simulink model "building_EXAMPLE_v1"  (R2016b)
settings: Solver=ode23tb  StartTime=-building.preruntime+8760*3600  StopTime=building.runtime+8760*3600  MaxStep=600  EnableMultiTasking=on
StartFcn:
  | tic
StopFcn:
  | toc
values from neighbouring files (symbols this model uses):
  building = create_building_automatic(building, modify, import_mode, name_XML, name_EXCEL, name_PHPP, NUMBEROFZONES)    [work_EXAMPLE_v1.m]
undefined symbols (not defined in the file or in its folder): A, B, C, cp, Dd, Dreifach, FluidMix, get_building, ID, MassFlow, p, Pressure, Qdot_C, Qdot_C_energy, Qdot_H, Qdot_H_energy, Qdot_I_electricity, Qdot_I_electricity_energy, Qdot_I_light, Qdot_I_light_energy, Qdot_I_person, Qdot_I_person_energy, Qdot_S, Qdot_S_energy, Qdot_T_ground, Qdot_T_ground_energy, Qdot_T_neighbour, Qdot_T_neighbour_energy, Qdot_T_opaque, Qdot_T_opaque_energy, Qdot_T_window, Qdot_T_window_energy, Qdot_V_infiltration, Qdot_V_infiltration_energy, Qdot_V_mech, Qdot_V_mech_energy, Qdot_V_window, Qdot_V_window_energy, rho, Tc, Temperature, Tr, Ts, Wärmeschutzglas, x_CO2, x_H2O, x_VOC
libraries: carnotUIBK x1931, carnot x83, simulink_extras x22, simulink x12
(part 13 of 35)

== system building_EXAMPLE_v1/HVAC pipes/ventilation_zone-to-zone 2-3 ==
  "[AIB]_in" : Inport
  "[AIB]_out" : Inport  Port=2
  Vdot : Inport  Port=3
  Bus Selector1 : BusSelector  OutputSignals=Tc,x_H2O,x_CO2,rho
  Bus Selector2 : BusSelector  OutputSignals=Tc,x_H2O,x_CO2,rho
  Demux5 : Demux  Outputs=2
  Fcn{1..4} (4 alike) : Fcn  Expr=u / (1+u)
  Gain : Gain  Gain=perc_Vdot_tot
  Gain{1,4..5,7} (4 alike) : Gain  Gain=-1
  Gain2 : Gain  Gain=0
  Ground{1..6,12..13} (8 alike) : Ground
  Mux1 : Mux  Inputs=[1 2 1 1 1 5 1 7]
  Mux2 : Mux  Inputs=[1 2 1 1 1 5 1 7]
  Mux3 : Mux  Inputs=2
  Mux6 : Mux  Inputs=2
  Product5 : Product  SaturateOnIntegerOverflow=on  InputSameDT=on  OutDataTypeStr=Inherit: Same as first input
  Product6 : Product  SaturateOnIntegerOverflow=on  InputSameDT=on  OutDataTypeStr=Inherit: Same as first input
  Product7 : Product  Inputs=3  SaturateOnIntegerOverflow=on  InputSameDT=on  OutDataTypeStr=Inherit: Same as first input
  Sum1 : Sum  Inputs=-+  SaturateOnIntegerOverflow=on  InputSameDT=on  OutDataTypeStr=Inherit: Same as first input
  Switch : Switch  Criteria=u2 > Threshold
  Switch1 : Switch  Criteria=u2 > Threshold
  cp : Constant  Value=1006.8
  h/s : Gain  Gain=1/3600
  "[S]_in" : Outport
  "[S]_out" : Outport  Port=2
  wires:
  Mux3/1 -> Switch1/1
  Mux6/1 -> Switch1/3
  Bus Selector1/3 -> Fcn3/1  "<x_CO2>"
  Bus Selector1/2 -> Fcn4/1  "<x_H2O>"
  Fcn3/1 -> Mux3/2
  Fcn4/1 -> Mux3/1
  Bus Selector2/4 -> Switch/3  "<rho>"
  Bus Selector1/4 -> Switch/1  "<rho>"
  "[AIB]_in"/1 -> Bus Selector1/1
  cp/1 -> Product7/3
  Ground4/1 -> Mux1/7
  Ground1/1 -> Mux1/8
  "[AIB]_out"/1 -> Bus Selector2/1
  Bus Selector1/1 -> Sum1/1  "<Tc>"
  Fcn1/1 -> Mux6/2
  Fcn2/1 -> Mux6/1
  Ground12/1 -> Mux1/6
  Product5/1 -> Demux5/1
  Bus Selector2/3 -> Fcn1/1  "<x_CO2>"
  Mux2/1 -> "[S]_out"/1
  Switch/1 -> Product6/2  "rho"
  Product6/1 -> Gain1/1
  Gain/1 -> Switch/2, Switch1/2, h/s/1
  Mux1/1 -> "[S]_in"/1
  Product7/1 -> Gain2/1, Mux1/1  "Qdot_air"
  Ground13/1 -> Mux1/2
  Demux5/2 -> Mux1/5, Gain5/1  "mdot_CO2"
  Demux5/1 -> Mux1/4, Gain4/1  "mdot_H2O"
  Bus Selector2/1 -> Sum1/2  "<Tc>"
  Bus Selector2/2 -> Fcn2/1  "<x_H2O>"
  Switch1/1 -> Product5/2
  Sum1/1 -> Product7/1  "dT"
  Vdot/1 -> Gain/1
  h/s/1 -> Product6/1
  Gain1/1 -> Gain7/1, Product5/1, Product7/2, Mux1/3  "massflow"
  Ground3/1 -> Mux2/7
  Gain4/1 -> Mux2/4
  Gain7/1 -> Mux2/3
  Ground2/1 -> Mux2/2
  Gain5/1 -> Mux2/5
  Ground5/1 -> Mux2/6
  Ground6/1 -> Mux2/8
  Gain2/1 -> Mux2/1

== system building_EXAMPLE_v1/HVAC pipes/ventilation_zone-to-zone 2-4 ==
  "[AIB]_in" : Inport
  "[AIB]_out" : Inport  Port=2
  Vdot : Inport  Port=3
  Bus Selector1 : BusSelector  OutputSignals=Tc,x_H2O,x_CO2,rho
  Bus Selector2 : BusSelector  OutputSignals=Tc,x_H2O,x_CO2,rho
  Demux5 : Demux  Outputs=2
  Fcn{1..4} (4 alike) : Fcn  Expr=u / (1+u)
  Gain : Gain  Gain=perc_Vdot_tot
  Gain{1,4..5,7} (4 alike) : Gain  Gain=-1
  Gain2 : Gain  Gain=0
  Ground{1..6,12..13} (8 alike) : Ground
  Mux1 : Mux  Inputs=[1 2 1 1 1 5 1 7]
  Mux2 : Mux  Inputs=[1 2 1 1 1 5 1 7]
  Mux3 : Mux  Inputs=2
  Mux6 : Mux  Inputs=2
  Product5 : Product  SaturateOnIntegerOverflow=on  InputSameDT=on  OutDataTypeStr=Inherit: Same as first input
  Product6 : Product  SaturateOnIntegerOverflow=on  InputSameDT=on  OutDataTypeStr=Inherit: Same as first input
  Product7 : Product  Inputs=3  SaturateOnIntegerOverflow=on  InputSameDT=on  OutDataTypeStr=Inherit: Same as first input
  Sum1 : Sum  Inputs=-+  SaturateOnIntegerOverflow=on  InputSameDT=on  OutDataTypeStr=Inherit: Same as first input
  Switch : Switch  Criteria=u2 > Threshold
  Switch1 : Switch  Criteria=u2 > Threshold
  cp : Constant  Value=1006.8
  h/s : Gain  Gain=1/3600
  "[S]_in" : Outport
  "[S]_out" : Outport  Port=2
  wires:
  Mux3/1 -> Switch1/1
  Mux6/1 -> Switch1/3
  Bus Selector1/3 -> Fcn3/1  "<x_CO2>"
  Bus Selector1/2 -> Fcn4/1  "<x_H2O>"
  Fcn3/1 -> Mux3/2
  Fcn4/1 -> Mux3/1
  Bus Selector2/4 -> Switch/3  "<rho>"
  Bus Selector1/4 -> Switch/1  "<rho>"
  "[AIB]_in"/1 -> Bus Selector1/1
  cp/1 -> Product7/3
  Ground4/1 -> Mux1/7
  Ground1/1 -> Mux1/8
  "[AIB]_out"/1 -> Bus Selector2/1
  Bus Selector1/1 -> Sum1/1  "<Tc>"
  Fcn1/1 -> Mux6/2
  Fcn2/1 -> Mux6/1
  Ground12/1 -> Mux1/6
  Product5/1 -> Demux5/1
  Bus Selector2/3 -> Fcn1/1  "<x_CO2>"
  Mux2/1 -> "[S]_out"/1
  Switch/1 -> Product6/2  "rho"
  Product6/1 -> Gain1/1
  Gain/1 -> Switch/2, Switch1/2, h/s/1
  Mux1/1 -> "[S]_in"/1
  Product7/1 -> Gain2/1, Mux1/1  "Qdot_air"
  Ground13/1 -> Mux1/2
  Demux5/2 -> Mux1/5, Gain5/1  "mdot_CO2"
  Demux5/1 -> Mux1/4, Gain4/1  "mdot_H2O"
  Bus Selector2/1 -> Sum1/2  "<Tc>"
  Bus Selector2/2 -> Fcn2/1  "<x_H2O>"
  Switch1/1 -> Product5/2
  Sum1/1 -> Product7/1  "dT"
  Vdot/1 -> Gain/1
  h/s/1 -> Product6/1
  Gain1/1 -> Gain7/1, Product5/1, Product7/2, Mux1/3  "massflow"
  Ground3/1 -> Mux2/7
  Gain4/1 -> Mux2/4
  Gain7/1 -> Mux2/3
  Ground2/1 -> Mux2/2
  Gain5/1 -> Mux2/5
  Ground5/1 -> Mux2/6
  Ground6/1 -> Mux2/8
  Gain2/1 -> Mux2/1

== system building_EXAMPLE_v1/HVAC pipes/ventilation_zone-to-zone 2-5 ==
  "[AIB]_in" : Inport
  "[AIB]_out" : Inport  Port=2
  Vdot : Inport  Port=3
  Bus Selector1 : BusSelector  OutputSignals=Tc,x_H2O,x_CO2,rho
  Bus Selector2 : BusSelector  OutputSignals=Tc,x_H2O,x_CO2,rho
  Demux5 : Demux  Outputs=2
  Fcn{1..4} (4 alike) : Fcn  Expr=u / (1+u)
  Gain : Gain  Gain=perc_Vdot_tot
  Gain{1,4..5,7} (4 alike) : Gain  Gain=-1
  Gain2 : Gain  Gain=0
  Ground{1..6,12..13} (8 alike) : Ground
  Mux1 : Mux  Inputs=[1 2 1 1 1 5 1 7]
  Mux2 : Mux  Inputs=[1 2 1 1 1 5 1 7]
  Mux3 : Mux  Inputs=2
  Mux6 : Mux  Inputs=2
  Product5 : Product  SaturateOnIntegerOverflow=on  InputSameDT=on  OutDataTypeStr=Inherit: Same as first input
  Product6 : Product  SaturateOnIntegerOverflow=on  InputSameDT=on  OutDataTypeStr=Inherit: Same as first input
  Product7 : Product  Inputs=3  SaturateOnIntegerOverflow=on  InputSameDT=on  OutDataTypeStr=Inherit: Same as first input
  Sum1 : Sum  Inputs=-+  SaturateOnIntegerOverflow=on  InputSameDT=on  OutDataTypeStr=Inherit: Same as first input
  Switch : Switch  Criteria=u2 > Threshold
  Switch1 : Switch  Criteria=u2 > Threshold
  cp : Constant  Value=1006.8
  h/s : Gain  Gain=1/3600
  "[S]_in" : Outport
  "[S]_out" : Outport  Port=2
  wires:
  Mux3/1 -> Switch1/1
  Mux6/1 -> Switch1/3
  Bus Selector1/3 -> Fcn3/1  "<x_CO2>"
  Bus Selector1/2 -> Fcn4/1  "<x_H2O>"
  Fcn3/1 -> Mux3/2
  Fcn4/1 -> Mux3/1
  Bus Selector2/4 -> Switch/3  "<rho>"
  Bus Selector1/4 -> Switch/1  "<rho>"
  "[AIB]_in"/1 -> Bus Selector1/1
  cp/1 -> Product7/3
  Ground4/1 -> Mux1/7
  Ground1/1 -> Mux1/8
  "[AIB]_out"/1 -> Bus Selector2/1
  Bus Selector1/1 -> Sum1/1  "<Tc>"
  Fcn1/1 -> Mux6/2
  Fcn2/1 -> Mux6/1
  Ground12/1 -> Mux1/6
  Product5/1 -> Demux5/1
  Bus Selector2/3 -> Fcn1/1  "<x_CO2>"
  Mux2/1 -> "[S]_out"/1
  Switch/1 -> Product6/2  "rho"
  Product6/1 -> Gain1/1
  Gain/1 -> Switch/2, Switch1/2, h/s/1
  Mux1/1 -> "[S]_in"/1
  Product7/1 -> Gain2/1, Mux1/1  "Qdot_air"
  Ground13/1 -> Mux1/2
  Demux5/2 -> Mux1/5, Gain5/1  "mdot_CO2"
  Demux5/1 -> Mux1/4, Gain4/1  "mdot_H2O"
  Bus Selector2/1 -> Sum1/2  "<Tc>"
  Bus Selector2/2 -> Fcn2/1  "<x_H2O>"
  Switch1/1 -> Product5/2
  Sum1/1 -> Product7/1  "dT"
  Vdot/1 -> Gain/1
  h/s/1 -> Product6/1
  Gain1/1 -> Gain7/1, Product5/1, Product7/2, Mux1/3  "massflow"
  Ground3/1 -> Mux2/7
  Gain4/1 -> Mux2/4
  Gain7/1 -> Mux2/3
  Ground2/1 -> Mux2/2
  Gain5/1 -> Mux2/5
  Ground5/1 -> Mux2/6
  Ground6/1 -> Mux2/8
  Gain2/1 -> Mux2/1

== system building_EXAMPLE_v1/HVAC pipes/ventilation_zone-to-zone 2-6 ==
  "[AIB]_in" : Inport
  "[AIB]_out" : Inport  Port=2
  Vdot : Inport  Port=3
  Bus Selector1 : BusSelector  OutputSignals=Tc,x_H2O,x_CO2,rho
  Bus Selector2 : BusSelector  OutputSignals=Tc,x_H2O,x_CO2,rho
  Demux5 : Demux  Outputs=2
  Fcn{1..4} (4 alike) : Fcn  Expr=u / (1+u)
  Gain : Gain  Gain=perc_Vdot_tot
  Gain{1,4..5,7} (4 alike) : Gain  Gain=-1
  Gain2 : Gain  Gain=0
  Ground{1..6,12..13} (8 alike) : Ground
  Mux1 : Mux  Inputs=[1 2 1 1 1 5 1 7]
  Mux2 : Mux  Inputs=[1 2 1 1 1 5 1 7]
  Mux3 : Mux  Inputs=2
  Mux6 : Mux  Inputs=2
  Product5 : Product  SaturateOnIntegerOverflow=on  InputSameDT=on  OutDataTypeStr=Inherit: Same as first input
  Product6 : Product  SaturateOnIntegerOverflow=on  InputSameDT=on  OutDataTypeStr=Inherit: Same as first input
  Product7 : Product  Inputs=3  SaturateOnIntegerOverflow=on  InputSameDT=on  OutDataTypeStr=Inherit: Same as first input
  Sum1 : Sum  Inputs=-+  SaturateOnIntegerOverflow=on  InputSameDT=on  OutDataTypeStr=Inherit: Same as first input
  Switch : Switch  Criteria=u2 > Threshold
  Switch1 : Switch  Criteria=u2 > Threshold
  cp : Constant  Value=1006.8
  h/s : Gain  Gain=1/3600
  "[S]_in" : Outport
  "[S]_out" : Outport  Port=2
  wires:
  Mux3/1 -> Switch1/1
  Mux6/1 -> Switch1/3
  Bus Selector1/3 -> Fcn3/1  "<x_CO2>"
  Bus Selector1/2 -> Fcn4/1  "<x_H2O>"
  Fcn3/1 -> Mux3/2
  Fcn4/1 -> Mux3/1
  Bus Selector2/4 -> Switch/3  "<rho>"
  Bus Selector1/4 -> Switch/1  "<rho>"
  "[AIB]_in"/1 -> Bus Selector1/1
  cp/1 -> Product7/3
  Ground4/1 -> Mux1/7
  Ground1/1 -> Mux1/8
  "[AIB]_out"/1 -> Bus Selector2/1
  Bus Selector1/1 -> Sum1/1  "<Tc>"
  Fcn1/1 -> Mux6/2
  Fcn2/1 -> Mux6/1
  Ground12/1 -> Mux1/6
  Product5/1 -> Demux5/1
  Bus Selector2/3 -> Fcn1/1  "<x_CO2>"
  Mux2/1 -> "[S]_out"/1
  Switch/1 -> Product6/2  "rho"
  Product6/1 -> Gain1/1
  Gain/1 -> Switch/2, Switch1/2, h/s/1
  Mux1/1 -> "[S]_in"/1
  Product7/1 -> Gain2/1, Mux1/1  "Qdot_air"
  Ground13/1 -> Mux1/2
  Demux5/2 -> Mux1/5, Gain5/1  "mdot_CO2"
  Demux5/1 -> Mux1/4, Gain4/1  "mdot_H2O"
  Bus Selector2/1 -> Sum1/2  "<Tc>"
  Bus Selector2/2 -> Fcn2/1  "<x_H2O>"
  Switch1/1 -> Product5/2
  Sum1/1 -> Product7/1  "dT"
  Vdot/1 -> Gain/1
  h/s/1 -> Product6/1
  Gain1/1 -> Gain7/1, Product5/1, Product7/2, Mux1/3  "massflow"
  Ground3/1 -> Mux2/7
  Gain4/1 -> Mux2/4
  Gain7/1 -> Mux2/3
  Ground2/1 -> Mux2/2
  Gain5/1 -> Mux2/5
  Ground5/1 -> Mux2/6
  Ground6/1 -> Mux2/8
  Gain2/1 -> Mux2/1

== system building_EXAMPLE_v1/HVAC pipes/ventilation_zone-to-zone 2-7 ==
  "[AIB]_in" : Inport
  "[AIB]_out" : Inport  Port=2
  Vdot : Inport  Port=3
  Bus Selector1 : BusSelector  OutputSignals=Tc,x_H2O,x_CO2,rho
  Bus Selector2 : BusSelector  OutputSignals=Tc,x_H2O,x_CO2,rho
  Demux5 : Demux  Outputs=2
  Fcn{1..4} (4 alike) : Fcn  Expr=u / (1+u)
  Gain : Gain  Gain=perc_Vdot_tot
  Gain{1,4..5,7} (4 alike) : Gain  Gain=-1
  Gain2 : Gain  Gain=0
  Ground{1..6,12..13} (8 alike) : Ground
  Mux1 : Mux  Inputs=[1 2 1 1 1 5 1 7]
  Mux2 : Mux  Inputs=[1 2 1 1 1 5 1 7]
  Mux3 : Mux  Inputs=2
  Mux6 : Mux  Inputs=2
  Product5 : Product  SaturateOnIntegerOverflow=on  InputSameDT=on  OutDataTypeStr=Inherit: Same as first input
  Product6 : Product  SaturateOnIntegerOverflow=on  InputSameDT=on  OutDataTypeStr=Inherit: Same as first input
  Product7 : Product  Inputs=3  SaturateOnIntegerOverflow=on  InputSameDT=on  OutDataTypeStr=Inherit: Same as first input
  Sum1 : Sum  Inputs=-+  SaturateOnIntegerOverflow=on  InputSameDT=on  OutDataTypeStr=Inherit: Same as first input
  Switch : Switch  Criteria=u2 > Threshold
  Switch1 : Switch  Criteria=u2 > Threshold
  cp : Constant  Value=1006.8
  h/s : Gain  Gain=1/3600
  "[S]_in" : Outport
  "[S]_out" : Outport  Port=2
  wires:
  Mux3/1 -> Switch1/1
  Mux6/1 -> Switch1/3
  Bus Selector1/3 -> Fcn3/1  "<x_CO2>"
  Bus Selector1/2 -> Fcn4/1  "<x_H2O>"
  Fcn3/1 -> Mux3/2
  Fcn4/1 -> Mux3/1
  Bus Selector2/4 -> Switch/3  "<rho>"
  Bus Selector1/4 -> Switch/1  "<rho>"
  "[AIB]_in"/1 -> Bus Selector1/1
  cp/1 -> Product7/3
  Ground4/1 -> Mux1/7
  Ground1/1 -> Mux1/8
  "[AIB]_out"/1 -> Bus Selector2/1
  Bus Selector1/1 -> Sum1/1  "<Tc>"
  Fcn1/1 -> Mux6/2
  Fcn2/1 -> Mux6/1
  Ground12/1 -> Mux1/6
  Product5/1 -> Demux5/1
  Bus Selector2/3 -> Fcn1/1  "<x_CO2>"
  Mux2/1 -> "[S]_out"/1
  Switch/1 -> Product6/2  "rho"
  Product6/1 -> Gain1/1
  Gain/1 -> Switch/2, Switch1/2, h/s/1
  Mux1/1 -> "[S]_in"/1
  Product7/1 -> Gain2/1, Mux1/1  "Qdot_air"
  Ground13/1 -> Mux1/2
  Demux5/2 -> Mux1/5, Gain5/1  "mdot_CO2"
  Demux5/1 -> Mux1/4, Gain4/1  "mdot_H2O"
  Bus Selector2/1 -> Sum1/2  "<Tc>"
  Bus Selector2/2 -> Fcn2/1  "<x_H2O>"
  Switch1/1 -> Product5/2
  Sum1/1 -> Product7/1  "dT"
  Vdot/1 -> Gain/1
  h/s/1 -> Product6/1
  Gain1/1 -> Gain7/1, Product5/1, Product7/2, Mux1/3  "massflow"
  Ground3/1 -> Mux2/7
  Gain4/1 -> Mux2/4
  Gain7/1 -> Mux2/3
  Ground2/1 -> Mux2/2
  Gain5/1 -> Mux2/5
  Ground5/1 -> Mux2/6
  Ground6/1 -> Mux2/8
  Gain2/1 -> Mux2/1

== system building_EXAMPLE_v1/HVAC pipes/ventilation_zone-to-zone 2-8 ==
  "[AIB]_in" : Inport
  "[AIB]_out" : Inport  Port=2
  Vdot : Inport  Port=3
  Bus Selector1 : BusSelector  OutputSignals=Tc,x_H2O,x_CO2,rho
  Bus Selector2 : BusSelector  OutputSignals=Tc,x_H2O,x_CO2,rho
  Demux5 : Demux  Outputs=2
  Fcn{1..4} (4 alike) : Fcn  Expr=u / (1+u)
  Gain : Gain  Gain=perc_Vdot_tot
  Gain{1,4..5,7} (4 alike) : Gain  Gain=-1
  Gain2 : Gain  Gain=0
  Ground{1..6,12..13} (8 alike) : Ground
  Mux1 : Mux  Inputs=[1 2 1 1 1 5 1 7]
  Mux2 : Mux  Inputs=[1 2 1 1 1 5 1 7]
  Mux3 : Mux  Inputs=2
  Mux6 : Mux  Inputs=2
  Product5 : Product  SaturateOnIntegerOverflow=on  InputSameDT=on  OutDataTypeStr=Inherit: Same as first input
  Product6 : Product  SaturateOnIntegerOverflow=on  InputSameDT=on  OutDataTypeStr=Inherit: Same as first input
  Product7 : Product  Inputs=3  SaturateOnIntegerOverflow=on  InputSameDT=on  OutDataTypeStr=Inherit: Same as first input
  Sum1 : Sum  Inputs=-+  SaturateOnIntegerOverflow=on  InputSameDT=on  OutDataTypeStr=Inherit: Same as first input
  Switch : Switch  Criteria=u2 > Threshold
  Switch1 : Switch  Criteria=u2 > Threshold
  cp : Constant  Value=1006.8
  h/s : Gain  Gain=1/3600
  "[S]_in" : Outport
  "[S]_out" : Outport  Port=2
  wires:
  Mux3/1 -> Switch1/1
  Mux6/1 -> Switch1/3
  Bus Selector1/3 -> Fcn3/1  "<x_CO2>"
  Bus Selector1/2 -> Fcn4/1  "<x_H2O>"
  Fcn3/1 -> Mux3/2
  Fcn4/1 -> Mux3/1
  Bus Selector2/4 -> Switch/3  "<rho>"
  Bus Selector1/4 -> Switch/1  "<rho>"
  "[AIB]_in"/1 -> Bus Selector1/1
  cp/1 -> Product7/3
  Ground4/1 -> Mux1/7
  Ground1/1 -> Mux1/8
  "[AIB]_out"/1 -> Bus Selector2/1
  Bus Selector1/1 -> Sum1/1  "<Tc>"
  Fcn1/1 -> Mux6/2
  Fcn2/1 -> Mux6/1
  Ground12/1 -> Mux1/6
  Product5/1 -> Demux5/1
  Bus Selector2/3 -> Fcn1/1  "<x_CO2>"
  Mux2/1 -> "[S]_out"/1
  Switch/1 -> Product6/2  "rho"
  Product6/1 -> Gain1/1
  Gain/1 -> Switch/2, Switch1/2, h/s/1
  Mux1/1 -> "[S]_in"/1
  Product7/1 -> Gain2/1, Mux1/1  "Qdot_air"
  Ground13/1 -> Mux1/2
  Demux5/2 -> Mux1/5, Gain5/1  "mdot_CO2"
  Demux5/1 -> Mux1/4, Gain4/1  "mdot_H2O"
  Bus Selector2/1 -> Sum1/2  "<Tc>"
  Bus Selector2/2 -> Fcn2/1  "<x_H2O>"
  Switch1/1 -> Product5/2
  Sum1/1 -> Product7/1  "dT"
  Vdot/1 -> Gain/1
  h/s/1 -> Product6/1
  Gain1/1 -> Gain7/1, Product5/1, Product7/2, Mux1/3  "massflow"
  Ground3/1 -> Mux2/7
  Gain4/1 -> Mux2/4
  Gain7/1 -> Mux2/3
  Ground2/1 -> Mux2/2
  Gain5/1 -> Mux2/5
  Ground5/1 -> Mux2/6
  Ground6/1 -> Mux2/8
  Gain2/1 -> Mux2/1

== system building_EXAMPLE_v1/HVAC pipes/ventilation_zone-to-zone 2-9 ==
  "[AIB]_in" : Inport
  "[AIB]_out" : Inport  Port=2
  Vdot : Inport  Port=3
  Bus Selector1 : BusSelector  OutputSignals=Tc,x_H2O,x_CO2,rho
  Bus Selector2 : BusSelector  OutputSignals=Tc,x_H2O,x_CO2,rho
  Demux5 : Demux  Outputs=2
  Fcn{1..4} (4 alike) : Fcn  Expr=u / (1+u)
  Gain : Gain  Gain=perc_Vdot_tot
  Gain{1,4..5,7} (4 alike) : Gain  Gain=-1
  Gain2 : Gain  Gain=0
  Ground{1..6,12..13} (8 alike) : Ground
  Mux1 : Mux  Inputs=[1 2 1 1 1 5 1 7]
  Mux2 : Mux  Inputs=[1 2 1 1 1 5 1 7]
  Mux3 : Mux  Inputs=2
  Mux6 : Mux  Inputs=2
  Product5 : Product  SaturateOnIntegerOverflow=on  InputSameDT=on  OutDataTypeStr=Inherit: Same as first input
  Product6 : Product  SaturateOnIntegerOverflow=on  InputSameDT=on  OutDataTypeStr=Inherit: Same as first input
  Product7 : Product  Inputs=3  SaturateOnIntegerOverflow=on  InputSameDT=on  OutDataTypeStr=Inherit: Same as first input
  Sum1 : Sum  Inputs=-+  SaturateOnIntegerOverflow=on  InputSameDT=on  OutDataTypeStr=Inherit: Same as first input
  Switch : Switch  Criteria=u2 > Threshold
  Switch1 : Switch  Criteria=u2 > Threshold
  cp : Constant  Value=1006.8
  h/s : Gain  Gain=1/3600
  "[S]_in" : Outport
  "[S]_out" : Outport  Port=2
  wires:
  Mux3/1 -> Switch1/1
  Mux6/1 -> Switch1/3
  Bus Selector1/3 -> Fcn3/1  "<x_CO2>"
  Bus Selector1/2 -> Fcn4/1  "<x_H2O>"
  Fcn3/1 -> Mux3/2
  Fcn4/1 -> Mux3/1
  Bus Selector2/4 -> Switch/3  "<rho>"
  Bus Selector1/4 -> Switch/1  "<rho>"
  "[AIB]_in"/1 -> Bus Selector1/1
  cp/1 -> Product7/3
  Ground4/1 -> Mux1/7
  Ground1/1 -> Mux1/8
  "[AIB]_out"/1 -> Bus Selector2/1
  Bus Selector1/1 -> Sum1/1  "<Tc>"
  Fcn1/1 -> Mux6/2
  Fcn2/1 -> Mux6/1
  Ground12/1 -> Mux1/6
  Product5/1 -> Demux5/1
  Bus Selector2/3 -> Fcn1/1  "<x_CO2>"
  Mux2/1 -> "[S]_out"/1
  Switch/1 -> Product6/2  "rho"
  Product6/1 -> Gain1/1
  Gain/1 -> Switch/2, Switch1/2, h/s/1
  Mux1/1 -> "[S]_in"/1
  Product7/1 -> Gain2/1, Mux1/1  "Qdot_air"
  Ground13/1 -> Mux1/2
  Demux5/2 -> Mux1/5, Gain5/1  "mdot_CO2"
  Demux5/1 -> Mux1/4, Gain4/1  "mdot_H2O"
  Bus Selector2/1 -> Sum1/2  "<Tc>"
  Bus Selector2/2 -> Fcn2/1  "<x_H2O>"
  Switch1/1 -> Product5/2
  Sum1/1 -> Product7/1  "dT"
  Vdot/1 -> Gain/1
  h/s/1 -> Product6/1
  Gain1/1 -> Gain7/1, Product5/1, Product7/2, Mux1/3  "massflow"
  Ground3/1 -> Mux2/7
  Gain4/1 -> Mux2/4
  Gain7/1 -> Mux2/3
  Ground2/1 -> Mux2/2
  Gain5/1 -> Mux2/5
  Ground5/1 -> Mux2/6
  Ground6/1 -> Mux2/8
  Gain2/1 -> Mux2/1

== system building_EXAMPLE_v1/HVAC pipes/ventilation_zone-to-zone 3-10 ==
  "[AIB]_in" : Inport
  "[AIB]_out" : Inport  Port=2
  Vdot : Inport  Port=3
  Bus Selector1 : BusSelector  OutputSignals=Tc,x_H2O,x_CO2,rho
  Bus Selector2 : BusSelector  OutputSignals=Tc,x_H2O,x_CO2,rho
  Demux5 : Demux  Outputs=2
  Fcn{1..4} (4 alike) : Fcn  Expr=u / (1+u)
  Gain : Gain  Gain=perc_Vdot_tot
  Gain{1,4..5,7} (4 alike) : Gain  Gain=-1
  Gain2 : Gain  Gain=0
  Ground{1..6,12..13} (8 alike) : Ground
  Mux1 : Mux  Inputs=[1 2 1 1 1 5 1 7]
  Mux2 : Mux  Inputs=[1 2 1 1 1 5 1 7]
  Mux3 : Mux  Inputs=2
  Mux6 : Mux  Inputs=2
  Product5 : Product  SaturateOnIntegerOverflow=on  InputSameDT=on  OutDataTypeStr=Inherit: Same as first input
  Product6 : Product  SaturateOnIntegerOverflow=on  InputSameDT=on  OutDataTypeStr=Inherit: Same as first input
  Product7 : Product  Inputs=3  SaturateOnIntegerOverflow=on  InputSameDT=on  OutDataTypeStr=Inherit: Same as first input
  Sum1 : Sum  Inputs=-+  SaturateOnIntegerOverflow=on  InputSameDT=on  OutDataTypeStr=Inherit: Same as first input
  Switch : Switch  Criteria=u2 > Threshold
  Switch1 : Switch  Criteria=u2 > Threshold
  cp : Constant  Value=1006.8
  h/s : Gain  Gain=1/3600
  "[S]_in" : Outport
  "[S]_out" : Outport  Port=2
  wires:
  Gain2/1 -> Mux2/1
  Ground6/1 -> Mux2/8
  Ground5/1 -> Mux2/6
  Gain5/1 -> Mux2/5
  Ground2/1 -> Mux2/2
  Gain7/1 -> Mux2/3
  Gain4/1 -> Mux2/4
  Ground3/1 -> Mux2/7
  Gain1/1 -> Mux1/3, Product7/2, Product5/1, Gain7/1  "massflow"
  h/s/1 -> Product6/1
  Vdot/1 -> Gain/1
  Sum1/1 -> Product7/1  "dT"
  Switch1/1 -> Product5/2
  Bus Selector2/2 -> Fcn2/1  "<x_H2O>"
  Bus Selector2/1 -> Sum1/2  "<Tc>"
  Demux5/1 -> Gain4/1, Mux1/4  "mdot_H2O"
  Demux5/2 -> Gain5/1, Mux1/5  "mdot_CO2"
  Ground13/1 -> Mux1/2
  Product7/1 -> Mux1/1, Gain2/1  "Qdot_air"
  Mux1/1 -> "[S]_in"/1
  Gain/1 -> h/s/1, Switch1/2, Switch/2
  Product6/1 -> Gain1/1
  Switch/1 -> Product6/2  "rho"
  Mux2/1 -> "[S]_out"/1
  Bus Selector2/3 -> Fcn1/1  "<x_CO2>"
  Product5/1 -> Demux5/1
  Ground12/1 -> Mux1/6
  Fcn2/1 -> Mux6/1
  Fcn1/1 -> Mux6/2
  Bus Selector1/1 -> Sum1/1  "<Tc>"
  "[AIB]_out"/1 -> Bus Selector2/1
  Ground1/1 -> Mux1/8
  Ground4/1 -> Mux1/7
  cp/1 -> Product7/3
  "[AIB]_in"/1 -> Bus Selector1/1
  Bus Selector1/4 -> Switch/1  "<rho>"
  Bus Selector2/4 -> Switch/3  "<rho>"
  Fcn4/1 -> Mux3/1
  Fcn3/1 -> Mux3/2
  Bus Selector1/2 -> Fcn4/1  "<x_H2O>"
  Bus Selector1/3 -> Fcn3/1  "<x_CO2>"
  Mux6/1 -> Switch1/3
  Mux3/1 -> Switch1/1

== system building_EXAMPLE_v1/HVAC pipes/ventilation_zone-to-zone 3-4 ==
  "[AIB]_in" : Inport
  "[AIB]_out" : Inport  Port=2
  Vdot : Inport  Port=3
  Bus Selector1 : BusSelector  OutputSignals=Tc,x_H2O,x_CO2,rho
  Bus Selector2 : BusSelector  OutputSignals=Tc,x_H2O,x_CO2,rho
  Demux5 : Demux  Outputs=2
  Fcn{1..4} (4 alike) : Fcn  Expr=u / (1+u)
  Gain : Gain  Gain=perc_Vdot_tot
  Gain{1,4..5,7} (4 alike) : Gain  Gain=-1
  Gain2 : Gain  Gain=0
  Ground{1..6,12..13} (8 alike) : Ground
  Mux1 : Mux  Inputs=[1 2 1 1 1 5 1 7]
  Mux2 : Mux  Inputs=[1 2 1 1 1 5 1 7]
  Mux3 : Mux  Inputs=2
  Mux6 : Mux  Inputs=2
  Product5 : Product  SaturateOnIntegerOverflow=on  InputSameDT=on  OutDataTypeStr=Inherit: Same as first input
  Product6 : Product  SaturateOnIntegerOverflow=on  InputSameDT=on  OutDataTypeStr=Inherit: Same as first input
  Product7 : Product  Inputs=3  SaturateOnIntegerOverflow=on  InputSameDT=on  OutDataTypeStr=Inherit: Same as first input
  Sum1 : Sum  Inputs=-+  SaturateOnIntegerOverflow=on  InputSameDT=on  OutDataTypeStr=Inherit: Same as first input
  Switch : Switch  Criteria=u2 > Threshold
  Switch1 : Switch  Criteria=u2 > Threshold
  cp : Constant  Value=1006.8
  h/s : Gain  Gain=1/3600
  "[S]_in" : Outport
  "[S]_out" : Outport  Port=2
  wires:
  Mux3/1 -> Switch1/1
  Mux6/1 -> Switch1/3
  Bus Selector1/3 -> Fcn3/1  "<x_CO2>"
  Bus Selector1/2 -> Fcn4/1  "<x_H2O>"
  Fcn3/1 -> Mux3/2
  Fcn4/1 -> Mux3/1
  Bus Selector2/4 -> Switch/3  "<rho>"
  Bus Selector1/4 -> Switch/1  "<rho>"
  "[AIB]_in"/1 -> Bus Selector1/1
  cp/1 -> Product7/3
  Ground4/1 -> Mux1/7
  Ground1/1 -> Mux1/8
  "[AIB]_out"/1 -> Bus Selector2/1
  Bus Selector1/1 -> Sum1/1  "<Tc>"
  Fcn1/1 -> Mux6/2
  Fcn2/1 -> Mux6/1
  Ground12/1 -> Mux1/6
  Product5/1 -> Demux5/1
  Bus Selector2/3 -> Fcn1/1  "<x_CO2>"
  Mux2/1 -> "[S]_out"/1
  Switch/1 -> Product6/2  "rho"
  Product6/1 -> Gain1/1
  Gain/1 -> Switch/2, Switch1/2, h/s/1
  Mux1/1 -> "[S]_in"/1
  Product7/1 -> Gain2/1, Mux1/1  "Qdot_air"
  Ground13/1 -> Mux1/2
  Demux5/2 -> Mux1/5, Gain5/1  "mdot_CO2"
  Demux5/1 -> Mux1/4, Gain4/1  "mdot_H2O"
  Bus Selector2/1 -> Sum1/2  "<Tc>"
  Bus Selector2/2 -> Fcn2/1  "<x_H2O>"
  Switch1/1 -> Product5/2
  Sum1/1 -> Product7/1  "dT"
  Vdot/1 -> Gain/1
  h/s/1 -> Product6/1
  Gain1/1 -> Gain7/1, Product5/1, Product7/2, Mux1/3  "massflow"
  Ground3/1 -> Mux2/7
  Gain4/1 -> Mux2/4
  Gain7/1 -> Mux2/3
  Ground2/1 -> Mux2/2
  Gain5/1 -> Mux2/5
  Ground5/1 -> Mux2/6
  Ground6/1 -> Mux2/8
  Gain2/1 -> Mux2/1

== system building_EXAMPLE_v1/HVAC pipes/ventilation_zone-to-zone 3-5 ==
  "[AIB]_in" : Inport
  "[AIB]_out" : Inport  Port=2
  Vdot : Inport  Port=3
  Bus Selector1 : BusSelector  OutputSignals=Tc,x_H2O,x_CO2,rho
  Bus Selector2 : BusSelector  OutputSignals=Tc,x_H2O,x_CO2,rho
  Demux5 : Demux  Outputs=2
  Fcn{1..4} (4 alike) : Fcn  Expr=u / (1+u)
  Gain : Gain  Gain=perc_Vdot_tot
  Gain{1,4..5,7} (4 alike) : Gain  Gain=-1
  Gain2 : Gain  Gain=0
  Ground{1..6,12..13} (8 alike) : Ground
  Mux1 : Mux  Inputs=[1 2 1 1 1 5 1 7]
  Mux2 : Mux  Inputs=[1 2 1 1 1 5 1 7]
  Mux3 : Mux  Inputs=2
  Mux6 : Mux  Inputs=2
  Product5 : Product  SaturateOnIntegerOverflow=on  InputSameDT=on  OutDataTypeStr=Inherit: Same as first input
  Product6 : Product  SaturateOnIntegerOverflow=on  InputSameDT=on  OutDataTypeStr=Inherit: Same as first input
  Product7 : Product  Inputs=3  SaturateOnIntegerOverflow=on  InputSameDT=on  OutDataTypeStr=Inherit: Same as first input
  Sum1 : Sum  Inputs=-+  SaturateOnIntegerOverflow=on  InputSameDT=on  OutDataTypeStr=Inherit: Same as first input
  Switch : Switch  Criteria=u2 > Threshold
  Switch1 : Switch  Criteria=u2 > Threshold
  cp : Constant  Value=1006.8
  h/s : Gain  Gain=1/3600
  "[S]_in" : Outport
  "[S]_out" : Outport  Port=2
  wires:
  Mux3/1 -> Switch1/1
  Mux6/1 -> Switch1/3
  Bus Selector1/3 -> Fcn3/1  "<x_CO2>"
  Bus Selector1/2 -> Fcn4/1  "<x_H2O>"
  Fcn3/1 -> Mux3/2
  Fcn4/1 -> Mux3/1
  Bus Selector2/4 -> Switch/3  "<rho>"
  Bus Selector1/4 -> Switch/1  "<rho>"
  "[AIB]_in"/1 -> Bus Selector1/1
  cp/1 -> Product7/3
  Ground4/1 -> Mux1/7
  Ground1/1 -> Mux1/8
  "[AIB]_out"/1 -> Bus Selector2/1
  Bus Selector1/1 -> Sum1/1  "<Tc>"
  Fcn1/1 -> Mux6/2
  Fcn2/1 -> Mux6/1
  Ground12/1 -> Mux1/6
  Product5/1 -> Demux5/1
  Bus Selector2/3 -> Fcn1/1  "<x_CO2>"
  Mux2/1 -> "[S]_out"/1
  Switch/1 -> Product6/2  "rho"
  Product6/1 -> Gain1/1
  Gain/1 -> Switch/2, Switch1/2, h/s/1
  Mux1/1 -> "[S]_in"/1
  Product7/1 -> Gain2/1, Mux1/1  "Qdot_air"
  Ground13/1 -> Mux1/2
  Demux5/2 -> Mux1/5, Gain5/1  "mdot_CO2"
  Demux5/1 -> Mux1/4, Gain4/1  "mdot_H2O"
  Bus Selector2/1 -> Sum1/2  "<Tc>"
  Bus Selector2/2 -> Fcn2/1  "<x_H2O>"
  Switch1/1 -> Product5/2
  Sum1/1 -> Product7/1  "dT"
  Vdot/1 -> Gain/1
  h/s/1 -> Product6/1
  Gain1/1 -> Gain7/1, Product5/1, Product7/2, Mux1/3  "massflow"
  Ground3/1 -> Mux2/7
  Gain4/1 -> Mux2/4
  Gain7/1 -> Mux2/3
  Ground2/1 -> Mux2/2
  Gain5/1 -> Mux2/5
  Ground5/1 -> Mux2/6
  Ground6/1 -> Mux2/8
  Gain2/1 -> Mux2/1

== system building_EXAMPLE_v1/HVAC pipes/ventilation_zone-to-zone 3-6 ==
  "[AIB]_in" : Inport
  "[AIB]_out" : Inport  Port=2
  Vdot : Inport  Port=3
  Bus Selector1 : BusSelector  OutputSignals=Tc,x_H2O,x_CO2,rho
  Bus Selector2 : BusSelector  OutputSignals=Tc,x_H2O,x_CO2,rho
  Demux5 : Demux  Outputs=2
  Fcn{1..4} (4 alike) : Fcn  Expr=u / (1+u)
  Gain : Gain  Gain=perc_Vdot_tot
  Gain{1,4..5,7} (4 alike) : Gain  Gain=-1
  Gain2 : Gain  Gain=0
  Ground{1..6,12..13} (8 alike) : Ground
  Mux1 : Mux  Inputs=[1 2 1 1 1 5 1 7]
  Mux2 : Mux  Inputs=[1 2 1 1 1 5 1 7]
  Mux3 : Mux  Inputs=2
  Mux6 : Mux  Inputs=2
  Product5 : Product  SaturateOnIntegerOverflow=on  InputSameDT=on  OutDataTypeStr=Inherit: Same as first input
  Product6 : Product  SaturateOnIntegerOverflow=on  InputSameDT=on  OutDataTypeStr=Inherit: Same as first input
  Product7 : Product  Inputs=3  SaturateOnIntegerOverflow=on  InputSameDT=on  OutDataTypeStr=Inherit: Same as first input
  Sum1 : Sum  Inputs=-+  SaturateOnIntegerOverflow=on  InputSameDT=on  OutDataTypeStr=Inherit: Same as first input
  Switch : Switch  Criteria=u2 > Threshold
  Switch1 : Switch  Criteria=u2 > Threshold
  cp : Constant  Value=1006.8
  h/s : Gain  Gain=1/3600
  "[S]_in" : Outport
  "[S]_out" : Outport  Port=2
  wires:
  Gain2/1 -> Mux2/1
  Ground6/1 -> Mux2/8
  Ground5/1 -> Mux2/6
  Gain5/1 -> Mux2/5
  Ground2/1 -> Mux2/2
  Gain7/1 -> Mux2/3
  Gain4/1 -> Mux2/4
  Ground3/1 -> Mux2/7
  Gain1/1 -> Mux1/3, Product7/2, Product5/1, Gain7/1  "massflow"
  h/s/1 -> Product6/1
  Vdot/1 -> Gain/1
  Sum1/1 -> Product7/1  "dT"
  Switch1/1 -> Product5/2
  Bus Selector2/2 -> Fcn2/1  "<x_H2O>"
  Bus Selector2/1 -> Sum1/2  "<Tc>"
  Demux5/1 -> Gain4/1, Mux1/4  "mdot_H2O"
  Demux5/2 -> Gain5/1, Mux1/5  "mdot_CO2"
  Ground13/1 -> Mux1/2
  Product7/1 -> Mux1/1, Gain2/1  "Qdot_air"
  Mux1/1 -> "[S]_in"/1
  Gain/1 -> h/s/1, Switch1/2, Switch/2
  Product6/1 -> Gain1/1
  Switch/1 -> Product6/2  "rho"
  Mux2/1 -> "[S]_out"/1
  Bus Selector2/3 -> Fcn1/1  "<x_CO2>"
  Product5/1 -> Demux5/1
  Ground12/1 -> Mux1/6
  Fcn2/1 -> Mux6/1
  Fcn1/1 -> Mux6/2
  Bus Selector1/1 -> Sum1/1  "<Tc>"
  "[AIB]_out"/1 -> Bus Selector2/1
  Ground1/1 -> Mux1/8
  Ground4/1 -> Mux1/7
  cp/1 -> Product7/3
  "[AIB]_in"/1 -> Bus Selector1/1
  Bus Selector1/4 -> Switch/1  "<rho>"
  Bus Selector2/4 -> Switch/3  "<rho>"
  Fcn4/1 -> Mux3/1
  Fcn3/1 -> Mux3/2
  Bus Selector1/2 -> Fcn4/1  "<x_H2O>"
  Bus Selector1/3 -> Fcn3/1  "<x_CO2>"
  Mux6/1 -> Switch1/3
  Mux3/1 -> Switch1/1

== system building_EXAMPLE_v1/HVAC pipes/ventilation_zone-to-zone 3-7 ==
  "[AIB]_in" : Inport
  "[AIB]_out" : Inport  Port=2
  Vdot : Inport  Port=3
  Bus Selector1 : BusSelector  OutputSignals=Tc,x_H2O,x_CO2,rho
  Bus Selector2 : BusSelector  OutputSignals=Tc,x_H2O,x_CO2,rho
  Demux5 : Demux  Outputs=2
  Fcn{1..4} (4 alike) : Fcn  Expr=u / (1+u)
  Gain : Gain  Gain=perc_Vdot_tot
  Gain{1,4..5,7} (4 alike) : Gain  Gain=-1
  Gain2 : Gain  Gain=0
  Ground{1..6,12..13} (8 alike) : Ground
  Mux1 : Mux  Inputs=[1 2 1 1 1 5 1 7]
  Mux2 : Mux  Inputs=[1 2 1 1 1 5 1 7]
  Mux3 : Mux  Inputs=2
  Mux6 : Mux  Inputs=2
  Product5 : Product  SaturateOnIntegerOverflow=on  InputSameDT=on  OutDataTypeStr=Inherit: Same as first input
  Product6 : Product  SaturateOnIntegerOverflow=on  InputSameDT=on  OutDataTypeStr=Inherit: Same as first input
  Product7 : Product  Inputs=3  SaturateOnIntegerOverflow=on  InputSameDT=on  OutDataTypeStr=Inherit: Same as first input
  Sum1 : Sum  Inputs=-+  SaturateOnIntegerOverflow=on  InputSameDT=on  OutDataTypeStr=Inherit: Same as first input
  Switch : Switch  Criteria=u2 > Threshold
  Switch1 : Switch  Criteria=u2 > Threshold
  cp : Constant  Value=1006.8
  h/s : Gain  Gain=1/3600
  "[S]_in" : Outport
  "[S]_out" : Outport  Port=2
  wires:
  Mux3/1 -> Switch1/1
  Mux6/1 -> Switch1/3
  Bus Selector1/3 -> Fcn3/1  "<x_CO2>"
  Bus Selector1/2 -> Fcn4/1  "<x_H2O>"
  Fcn3/1 -> Mux3/2
  Fcn4/1 -> Mux3/1
  Bus Selector2/4 -> Switch/3  "<rho>"
  Bus Selector1/4 -> Switch/1  "<rho>"
  "[AIB]_in"/1 -> Bus Selector1/1
  cp/1 -> Product7/3
  Ground4/1 -> Mux1/7
  Ground1/1 -> Mux1/8
  "[AIB]_out"/1 -> Bus Selector2/1
  Bus Selector1/1 -> Sum1/1  "<Tc>"
  Fcn1/1 -> Mux6/2
  Fcn2/1 -> Mux6/1
  Ground12/1 -> Mux1/6
  Product5/1 -> Demux5/1
  Bus Selector2/3 -> Fcn1/1  "<x_CO2>"
  Mux2/1 -> "[S]_out"/1
  Switch/1 -> Product6/2  "rho"
  Product6/1 -> Gain1/1
  Gain/1 -> Switch/2, Switch1/2, h/s/1
  Mux1/1 -> "[S]_in"/1
  Product7/1 -> Gain2/1, Mux1/1  "Qdot_air"
  Ground13/1 -> Mux1/2
  Demux5/2 -> Mux1/5, Gain5/1  "mdot_CO2"
  Demux5/1 -> Mux1/4, Gain4/1  "mdot_H2O"
  Bus Selector2/1 -> Sum1/2  "<Tc>"
  Bus Selector2/2 -> Fcn2/1  "<x_H2O>"
  Switch1/1 -> Product5/2
  Sum1/1 -> Product7/1  "dT"
  Vdot/1 -> Gain/1
  h/s/1 -> Product6/1
  Gain1/1 -> Gain7/1, Product5/1, Product7/2, Mux1/3  "massflow"
  Ground3/1 -> Mux2/7
  Gain4/1 -> Mux2/4
  Gain7/1 -> Mux2/3
  Ground2/1 -> Mux2/2
  Gain5/1 -> Mux2/5
  Ground5/1 -> Mux2/6
  Ground6/1 -> Mux2/8
  Gain2/1 -> Mux2/1

== system building_EXAMPLE_v1/HVAC pipes/ventilation_zone-to-zone 3-8 ==
  "[AIB]_in" : Inport
  "[AIB]_out" : Inport  Port=2
  Vdot : Inport  Port=3
  Bus Selector1 : BusSelector  OutputSignals=Tc,x_H2O,x_CO2,rho
  Bus Selector2 : BusSelector  OutputSignals=Tc,x_H2O,x_CO2,rho
  Demux5 : Demux  Outputs=2
  Fcn{1..4} (4 alike) : Fcn  Expr=u / (1+u)
  Gain : Gain  Gain=perc_Vdot_tot
  Gain{1,4..5,7} (4 alike) : Gain  Gain=-1
  Gain2 : Gain  Gain=0
  Ground{1..6,12..13} (8 alike) : Ground
  Mux1 : Mux  Inputs=[1 2 1 1 1 5 1 7]
  Mux2 : Mux  Inputs=[1 2 1 1 1 5 1 7]
  Mux3 : Mux  Inputs=2
  Mux6 : Mux  Inputs=2
  Product5 : Product  SaturateOnIntegerOverflow=on  InputSameDT=on  OutDataTypeStr=Inherit: Same as first input
  Product6 : Product  SaturateOnIntegerOverflow=on  InputSameDT=on  OutDataTypeStr=Inherit: Same as first input
  Product7 : Product  Inputs=3  SaturateOnIntegerOverflow=on  InputSameDT=on  OutDataTypeStr=Inherit: Same as first input
  Sum1 : Sum  Inputs=-+  SaturateOnIntegerOverflow=on  InputSameDT=on  OutDataTypeStr=Inherit: Same as first input
  Switch : Switch  Criteria=u2 > Threshold
  Switch1 : Switch  Criteria=u2 > Threshold
  cp : Constant  Value=1006.8
  h/s : Gain  Gain=1/3600
  "[S]_in" : Outport
  "[S]_out" : Outport  Port=2
  wires:
  Gain2/1 -> Mux2/1
  Ground6/1 -> Mux2/8
  Ground5/1 -> Mux2/6
  Gain5/1 -> Mux2/5
  Ground2/1 -> Mux2/2
  Gain7/1 -> Mux2/3
  Gain4/1 -> Mux2/4
  Ground3/1 -> Mux2/7
  Gain1/1 -> Mux1/3, Product7/2, Product5/1, Gain7/1  "massflow"
  h/s/1 -> Product6/1
  Vdot/1 -> Gain/1
  Sum1/1 -> Product7/1  "dT"
  Switch1/1 -> Product5/2
  Bus Selector2/2 -> Fcn2/1  "<x_H2O>"
  Bus Selector2/1 -> Sum1/2  "<Tc>"
  Demux5/1 -> Gain4/1, Mux1/4  "mdot_H2O"
  Demux5/2 -> Gain5/1, Mux1/5  "mdot_CO2"
  Ground13/1 -> Mux1/2
  Product7/1 -> Mux1/1, Gain2/1  "Qdot_air"
  Mux1/1 -> "[S]_in"/1
  Gain/1 -> h/s/1, Switch1/2, Switch/2
  Product6/1 -> Gain1/1
  Switch/1 -> Product6/2  "rho"
  Mux2/1 -> "[S]_out"/1
  Bus Selector2/3 -> Fcn1/1  "<x_CO2>"
  Product5/1 -> Demux5/1
  Ground12/1 -> Mux1/6
  Fcn2/1 -> Mux6/1
  Fcn1/1 -> Mux6/2
  Bus Selector1/1 -> Sum1/1  "<Tc>"
  "[AIB]_out"/1 -> Bus Selector2/1
  Ground1/1 -> Mux1/8
  Ground4/1 -> Mux1/7
  cp/1 -> Product7/3
  "[AIB]_in"/1 -> Bus Selector1/1
  Bus Selector1/4 -> Switch/1  "<rho>"
  Bus Selector2/4 -> Switch/3  "<rho>"
  Fcn4/1 -> Mux3/1
  Fcn3/1 -> Mux3/2
  Bus Selector1/2 -> Fcn4/1  "<x_H2O>"
  Bus Selector1/3 -> Fcn3/1  "<x_CO2>"
  Mux6/1 -> Switch1/3
  Mux3/1 -> Switch1/1

== system building_EXAMPLE_v1/HVAC pipes/ventilation_zone-to-zone 3-9 ==
  "[AIB]_in" : Inport
  "[AIB]_out" : Inport  Port=2
  Vdot : Inport  Port=3
  Bus Selector1 : BusSelector  OutputSignals=Tc,x_H2O,x_CO2,rho
  Bus Selector2 : BusSelector  OutputSignals=Tc,x_H2O,x_CO2,rho
  Demux5 : Demux  Outputs=2
  Fcn{1..4} (4 alike) : Fcn  Expr=u / (1+u)
  Gain : Gain  Gain=perc_Vdot_tot
  Gain{1,4..5,7} (4 alike) : Gain  Gain=-1
  Gain2 : Gain  Gain=0
  Ground{1..6,12..13} (8 alike) : Ground
  Mux1 : Mux  Inputs=[1 2 1 1 1 5 1 7]
  Mux2 : Mux  Inputs=[1 2 1 1 1 5 1 7]
  Mux3 : Mux  Inputs=2
  Mux6 : Mux  Inputs=2
  Product5 : Product  SaturateOnIntegerOverflow=on  InputSameDT=on  OutDataTypeStr=Inherit: Same as first input
  Product6 : Product  SaturateOnIntegerOverflow=on  InputSameDT=on  OutDataTypeStr=Inherit: Same as first input
  Product7 : Product  Inputs=3  SaturateOnIntegerOverflow=on  InputSameDT=on  OutDataTypeStr=Inherit: Same as first input
  Sum1 : Sum  Inputs=-+  SaturateOnIntegerOverflow=on  InputSameDT=on  OutDataTypeStr=Inherit: Same as first input
  Switch : Switch  Criteria=u2 > Threshold
  Switch1 : Switch  Criteria=u2 > Threshold
  cp : Constant  Value=1006.8
  h/s : Gain  Gain=1/3600
  "[S]_in" : Outport
  "[S]_out" : Outport  Port=2
  wires:
  Mux3/1 -> Switch1/1
  Mux6/1 -> Switch1/3
  Bus Selector1/3 -> Fcn3/1  "<x_CO2>"
  Bus Selector1/2 -> Fcn4/1  "<x_H2O>"
  Fcn3/1 -> Mux3/2
  Fcn4/1 -> Mux3/1
  Bus Selector2/4 -> Switch/3  "<rho>"
  Bus Selector1/4 -> Switch/1  "<rho>"
  "[AIB]_in"/1 -> Bus Selector1/1
  cp/1 -> Product7/3
  Ground4/1 -> Mux1/7
  Ground1/1 -> Mux1/8
  "[AIB]_out"/1 -> Bus Selector2/1
  Bus Selector1/1 -> Sum1/1  "<Tc>"
  Fcn1/1 -> Mux6/2
  Fcn2/1 -> Mux6/1
  Ground12/1 -> Mux1/6
  Product5/1 -> Demux5/1
  Bus Selector2/3 -> Fcn1/1  "<x_CO2>"
  Mux2/1 -> "[S]_out"/1
  Switch/1 -> Product6/2  "rho"
  Product6/1 -> Gain1/1
  Gain/1 -> Switch/2, Switch1/2, h/s/1
  Mux1/1 -> "[S]_in"/1
  Product7/1 -> Gain2/1, Mux1/1  "Qdot_air"
  Ground13/1 -> Mux1/2
  Demux5/2 -> Mux1/5, Gain5/1  "mdot_CO2"
  Demux5/1 -> Mux1/4, Gain4/1  "mdot_H2O"
  Bus Selector2/1 -> Sum1/2  "<Tc>"
  Bus Selector2/2 -> Fcn2/1  "<x_H2O>"
  Switch1/1 -> Product5/2
  Sum1/1 -> Product7/1  "dT"
  Vdot/1 -> Gain/1
  h/s/1 -> Product6/1
  Gain1/1 -> Gain7/1, Product5/1, Product7/2, Mux1/3  "massflow"
  Ground3/1 -> Mux2/7
  Gain4/1 -> Mux2/4
  Gain7/1 -> Mux2/3
  Ground2/1 -> Mux2/2
  Gain5/1 -> Mux2/5
  Ground5/1 -> Mux2/6
  Ground6/1 -> Mux2/8
  Gain2/1 -> Mux2/1

== system building_EXAMPLE_v1/HVAC pipes/ventilation_zone-to-zone 4-10 ==
  "[AIB]_in" : Inport
  "[AIB]_out" : Inport  Port=2
  Vdot : Inport  Port=3
  Bus Selector1 : BusSelector  OutputSignals=Tc,x_H2O,x_CO2,rho
  Bus Selector2 : BusSelector  OutputSignals=Tc,x_H2O,x_CO2,rho
  Demux5 : Demux  Outputs=2
  Fcn{1..4} (4 alike) : Fcn  Expr=u / (1+u)
  Gain : Gain  Gain=perc_Vdot_tot
  Gain{1,4..5,7} (4 alike) : Gain  Gain=-1
  Gain2 : Gain  Gain=0
  Ground{1..6,12..13} (8 alike) : Ground
  Mux1 : Mux  Inputs=[1 2 1 1 1 5 1 7]
  Mux2 : Mux  Inputs=[1 2 1 1 1 5 1 7]
  Mux3 : Mux  Inputs=2
  Mux6 : Mux  Inputs=2
  Product5 : Product  SaturateOnIntegerOverflow=on  InputSameDT=on  OutDataTypeStr=Inherit: Same as first input
  Product6 : Product  SaturateOnIntegerOverflow=on  InputSameDT=on  OutDataTypeStr=Inherit: Same as first input
  Product7 : Product  Inputs=3  SaturateOnIntegerOverflow=on  InputSameDT=on  OutDataTypeStr=Inherit: Same as first input
  Sum1 : Sum  Inputs=-+  SaturateOnIntegerOverflow=on  InputSameDT=on  OutDataTypeStr=Inherit: Same as first input
  Switch : Switch  Criteria=u2 > Threshold
  Switch1 : Switch  Criteria=u2 > Threshold
  cp : Constant  Value=1006.8
  h/s : Gain  Gain=1/3600
  "[S]_in" : Outport
  "[S]_out" : Outport  Port=2
  wires:
  Gain2/1 -> Mux2/1
  Ground6/1 -> Mux2/8
  Ground5/1 -> Mux2/6
  Gain5/1 -> Mux2/5
  Ground2/1 -> Mux2/2
  Gain7/1 -> Mux2/3
  Gain4/1 -> Mux2/4
  Ground3/1 -> Mux2/7
  Gain1/1 -> Mux1/3, Product7/2, Product5/1, Gain7/1  "massflow"
  h/s/1 -> Product6/1
  Vdot/1 -> Gain/1
  Sum1/1 -> Product7/1  "dT"
  Switch1/1 -> Product5/2
  Bus Selector2/2 -> Fcn2/1  "<x_H2O>"
  Bus Selector2/1 -> Sum1/2  "<Tc>"
  Demux5/1 -> Gain4/1, Mux1/4  "mdot_H2O"
  Demux5/2 -> Gain5/1, Mux1/5  "mdot_CO2"
  Ground13/1 -> Mux1/2
  Product7/1 -> Mux1/1, Gain2/1  "Qdot_air"
  Mux1/1 -> "[S]_in"/1
  Gain/1 -> h/s/1, Switch1/2, Switch/2
  Product6/1 -> Gain1/1
  Switch/1 -> Product6/2  "rho"
  Mux2/1 -> "[S]_out"/1
  Bus Selector2/3 -> Fcn1/1  "<x_CO2>"
  Product5/1 -> Demux5/1
  Ground12/1 -> Mux1/6
  Fcn2/1 -> Mux6/1
  Fcn1/1 -> Mux6/2
  Bus Selector1/1 -> Sum1/1  "<Tc>"
  "[AIB]_out"/1 -> Bus Selector2/1
  Ground1/1 -> Mux1/8
  Ground4/1 -> Mux1/7
  cp/1 -> Product7/3
  "[AIB]_in"/1 -> Bus Selector1/1
  Bus Selector1/4 -> Switch/1  "<rho>"
  Bus Selector2/4 -> Switch/3  "<rho>"
  Fcn4/1 -> Mux3/1
  Fcn3/1 -> Mux3/2
  Bus Selector1/2 -> Fcn4/1  "<x_H2O>"
  Bus Selector1/3 -> Fcn3/1  "<x_CO2>"
  Mux6/1 -> Switch1/3
  Mux3/1 -> Switch1/1

== system building_EXAMPLE_v1/HVAC pipes/ventilation_zone-to-zone 4-5 ==
  "[AIB]_in" : Inport
  "[AIB]_out" : Inport  Port=2
  Vdot : Inport  Port=3
  Bus Selector1 : BusSelector  OutputSignals=Tc,x_H2O,x_CO2,rho
  Bus Selector2 : BusSelector  OutputSignals=Tc,x_H2O,x_CO2,rho
  Demux5 : Demux  Outputs=2
  Fcn{1..4} (4 alike) : Fcn  Expr=u / (1+u)
  Gain : Gain  Gain=perc_Vdot_tot
  Gain{1,4..5,7} (4 alike) : Gain  Gain=-1
  Gain2 : Gain  Gain=0
  Ground{1..6,12..13} (8 alike) : Ground
  Mux1 : Mux  Inputs=[1 2 1 1 1 5 1 7]
  Mux2 : Mux  Inputs=[1 2 1 1 1 5 1 7]
  Mux3 : Mux  Inputs=2
  Mux6 : Mux  Inputs=2
  Product5 : Product  SaturateOnIntegerOverflow=on  InputSameDT=on  OutDataTypeStr=Inherit: Same as first input
  Product6 : Product  SaturateOnIntegerOverflow=on  InputSameDT=on  OutDataTypeStr=Inherit: Same as first input
  Product7 : Product  Inputs=3  SaturateOnIntegerOverflow=on  InputSameDT=on  OutDataTypeStr=Inherit: Same as first input
  Sum1 : Sum  Inputs=-+  SaturateOnIntegerOverflow=on  InputSameDT=on  OutDataTypeStr=Inherit: Same as first input
  Switch : Switch  Criteria=u2 > Threshold
  Switch1 : Switch  Criteria=u2 > Threshold
  cp : Constant  Value=1006.8
  h/s : Gain  Gain=1/3600
  "[S]_in" : Outport
  "[S]_out" : Outport  Port=2
  wires:
  Mux3/1 -> Switch1/1
  Mux6/1 -> Switch1/3
  Bus Selector1/3 -> Fcn3/1  "<x_CO2>"
  Bus Selector1/2 -> Fcn4/1  "<x_H2O>"
  Fcn3/1 -> Mux3/2
  Fcn4/1 -> Mux3/1
  Bus Selector2/4 -> Switch/3  "<rho>"
  Bus Selector1/4 -> Switch/1  "<rho>"
  "[AIB]_in"/1 -> Bus Selector1/1
  cp/1 -> Product7/3
  Ground4/1 -> Mux1/7
  Ground1/1 -> Mux1/8
  "[AIB]_out"/1 -> Bus Selector2/1
  Bus Selector1/1 -> Sum1/1  "<Tc>"
  Fcn1/1 -> Mux6/2
  Fcn2/1 -> Mux6/1
  Ground12/1 -> Mux1/6
  Product5/1 -> Demux5/1
  Bus Selector2/3 -> Fcn1/1  "<x_CO2>"
  Mux2/1 -> "[S]_out"/1
  Switch/1 -> Product6/2  "rho"
  Product6/1 -> Gain1/1
  Gain/1 -> Switch/2, Switch1/2, h/s/1
  Mux1/1 -> "[S]_in"/1
  Product7/1 -> Gain2/1, Mux1/1  "Qdot_air"
  Ground13/1 -> Mux1/2
  Demux5/2 -> Mux1/5, Gain5/1  "mdot_CO2"
  Demux5/1 -> Mux1/4, Gain4/1  "mdot_H2O"
  Bus Selector2/1 -> Sum1/2  "<Tc>"
  Bus Selector2/2 -> Fcn2/1  "<x_H2O>"
  Switch1/1 -> Product5/2
  Sum1/1 -> Product7/1  "dT"
  Vdot/1 -> Gain/1
  h/s/1 -> Product6/1
  Gain1/1 -> Gain7/1, Product5/1, Product7/2, Mux1/3  "massflow"
  Ground3/1 -> Mux2/7
  Gain4/1 -> Mux2/4
  Gain7/1 -> Mux2/3
  Ground2/1 -> Mux2/2
  Gain5/1 -> Mux2/5
  Ground5/1 -> Mux2/6
  Ground6/1 -> Mux2/8
  Gain2/1 -> Mux2/1

== system building_EXAMPLE_v1/HVAC pipes/ventilation_zone-to-zone 4-6 ==
  "[AIB]_in" : Inport
  "[AIB]_out" : Inport  Port=2
  Vdot : Inport  Port=3
  Bus Selector1 : BusSelector  OutputSignals=Tc,x_H2O,x_CO2,rho
  Bus Selector2 : BusSelector  OutputSignals=Tc,x_H2O,x_CO2,rho
  Demux5 : Demux  Outputs=2
  Fcn{1..4} (4 alike) : Fcn  Expr=u / (1+u)
  Gain : Gain  Gain=perc_Vdot_tot
  Gain{1,4..5,7} (4 alike) : Gain  Gain=-1
  Gain2 : Gain  Gain=0
  Ground{1..6,12..13} (8 alike) : Ground
  Mux1 : Mux  Inputs=[1 2 1 1 1 5 1 7]
  Mux2 : Mux  Inputs=[1 2 1 1 1 5 1 7]
  Mux3 : Mux  Inputs=2
  Mux6 : Mux  Inputs=2
  Product5 : Product  SaturateOnIntegerOverflow=on  InputSameDT=on  OutDataTypeStr=Inherit: Same as first input
  Product6 : Product  SaturateOnIntegerOverflow=on  InputSameDT=on  OutDataTypeStr=Inherit: Same as first input
  Product7 : Product  Inputs=3  SaturateOnIntegerOverflow=on  InputSameDT=on  OutDataTypeStr=Inherit: Same as first input
  Sum1 : Sum  Inputs=-+  SaturateOnIntegerOverflow=on  InputSameDT=on  OutDataTypeStr=Inherit: Same as first input
  Switch : Switch  Criteria=u2 > Threshold
  Switch1 : Switch  Criteria=u2 > Threshold
  cp : Constant  Value=1006.8
  h/s : Gain  Gain=1/3600
  "[S]_in" : Outport
  "[S]_out" : Outport  Port=2
  wires:
  Gain2/1 -> Mux2/1
  Ground6/1 -> Mux2/8
  Ground5/1 -> Mux2/6
  Gain5/1 -> Mux2/5
  Ground2/1 -> Mux2/2
  Gain7/1 -> Mux2/3
  Gain4/1 -> Mux2/4
  Ground3/1 -> Mux2/7
  Gain1/1 -> Mux1/3, Product7/2, Product5/1, Gain7/1  "massflow"
  h/s/1 -> Product6/1
  Vdot/1 -> Gain/1
  Sum1/1 -> Product7/1  "dT"
  Switch1/1 -> Product5/2
  Bus Selector2/2 -> Fcn2/1  "<x_H2O>"
  Bus Selector2/1 -> Sum1/2  "<Tc>"
  Demux5/1 -> Gain4/1, Mux1/4  "mdot_H2O"
  Demux5/2 -> Gain5/1, Mux1/5  "mdot_CO2"
  Ground13/1 -> Mux1/2
  Product7/1 -> Mux1/1, Gain2/1  "Qdot_air"
  Mux1/1 -> "[S]_in"/1
  Gain/1 -> h/s/1, Switch1/2, Switch/2
  Product6/1 -> Gain1/1
  Switch/1 -> Product6/2  "rho"
  Mux2/1 -> "[S]_out"/1
  Bus Selector2/3 -> Fcn1/1  "<x_CO2>"
  Product5/1 -> Demux5/1
  Ground12/1 -> Mux1/6
  Fcn2/1 -> Mux6/1
  Fcn1/1 -> Mux6/2
  Bus Selector1/1 -> Sum1/1  "<Tc>"
  "[AIB]_out"/1 -> Bus Selector2/1
  Ground1/1 -> Mux1/8
  Ground4/1 -> Mux1/7
  cp/1 -> Product7/3
  "[AIB]_in"/1 -> Bus Selector1/1
  Bus Selector1/4 -> Switch/1  "<rho>"
  Bus Selector2/4 -> Switch/3  "<rho>"
  Fcn4/1 -> Mux3/1
  Fcn3/1 -> Mux3/2
  Bus Selector1/2 -> Fcn4/1  "<x_H2O>"
  Bus Selector1/3 -> Fcn3/1  "<x_CO2>"
  Mux6/1 -> Switch1/3
  Mux3/1 -> Switch1/1

== system building_EXAMPLE_v1/HVAC pipes/ventilation_zone-to-zone 4-7 ==
  "[AIB]_in" : Inport
  "[AIB]_out" : Inport  Port=2
  Vdot : Inport  Port=3
  Bus Selector1 : BusSelector  OutputSignals=Tc,x_H2O,x_CO2,rho
  Bus Selector2 : BusSelector  OutputSignals=Tc,x_H2O,x_CO2,rho
  Demux5 : Demux  Outputs=2
  Fcn{1..4} (4 alike) : Fcn  Expr=u / (1+u)
  Gain : Gain  Gain=perc_Vdot_tot
  Gain{1,4..5,7} (4 alike) : Gain  Gain=-1
  Gain2 : Gain  Gain=0
  Ground{1..6,12..13} (8 alike) : Ground
  Mux1 : Mux  Inputs=[1 2 1 1 1 5 1 7]
  Mux2 : Mux  Inputs=[1 2 1 1 1 5 1 7]
  Mux3 : Mux  Inputs=2
  Mux6 : Mux  Inputs=2
  Product5 : Product  SaturateOnIntegerOverflow=on  InputSameDT=on  OutDataTypeStr=Inherit: Same as first input
  Product6 : Product  SaturateOnIntegerOverflow=on  InputSameDT=on  OutDataTypeStr=Inherit: Same as first input
  Product7 : Product  Inputs=3  SaturateOnIntegerOverflow=on  InputSameDT=on  OutDataTypeStr=Inherit: Same as first input
  Sum1 : Sum  Inputs=-+  SaturateOnIntegerOverflow=on  InputSameDT=on  OutDataTypeStr=Inherit: Same as first input
  Switch : Switch  Criteria=u2 > Threshold
  Switch1 : Switch  Criteria=u2 > Threshold
  cp : Constant  Value=1006.8
  h/s : Gain  Gain=1/3600
  "[S]_in" : Outport
  "[S]_out" : Outport  Port=2
  wires:
  Mux3/1 -> Switch1/1
  Mux6/1 -> Switch1/3
  Bus Selector1/3 -> Fcn3/1  "<x_CO2>"
  Bus Selector1/2 -> Fcn4/1  "<x_H2O>"
  Fcn3/1 -> Mux3/2
  Fcn4/1 -> Mux3/1
  Bus Selector2/4 -> Switch/3  "<rho>"
  Bus Selector1/4 -> Switch/1  "<rho>"
  "[AIB]_in"/1 -> Bus Selector1/1
  cp/1 -> Product7/3
  Ground4/1 -> Mux1/7
  Ground1/1 -> Mux1/8
  "[AIB]_out"/1 -> Bus Selector2/1
  Bus Selector1/1 -> Sum1/1  "<Tc>"
  Fcn1/1 -> Mux6/2
  Fcn2/1 -> Mux6/1
  Ground12/1 -> Mux1/6
  Product5/1 -> Demux5/1
  Bus Selector2/3 -> Fcn1/1  "<x_CO2>"
  Mux2/1 -> "[S]_out"/1
  Switch/1 -> Product6/2  "rho"
  Product6/1 -> Gain1/1
  Gain/1 -> Switch/2, Switch1/2, h/s/1
  Mux1/1 -> "[S]_in"/1
  Product7/1 -> Gain2/1, Mux1/1  "Qdot_air"
  Ground13/1 -> Mux1/2
  Demux5/2 -> Mux1/5, Gain5/1  "mdot_CO2"
  Demux5/1 -> Mux1/4, Gain4/1  "mdot_H2O"
  Bus Selector2/1 -> Sum1/2  "<Tc>"
  Bus Selector2/2 -> Fcn2/1  "<x_H2O>"
  Switch1/1 -> Product5/2
  Sum1/1 -> Product7/1  "dT"
  Vdot/1 -> Gain/1
  h/s/1 -> Product6/1
  Gain1/1 -> Gain7/1, Product5/1, Product7/2, Mux1/3  "massflow"
  Ground3/1 -> Mux2/7
  Gain4/1 -> Mux2/4
  Gain7/1 -> Mux2/3
  Ground2/1 -> Mux2/2
  Gain5/1 -> Mux2/5
  Ground5/1 -> Mux2/6
  Ground6/1 -> Mux2/8
  Gain2/1 -> Mux2/1

== system building_EXAMPLE_v1/HVAC pipes/ventilation_zone-to-zone 4-8 ==
  "[AIB]_in" : Inport
  "[AIB]_out" : Inport  Port=2
  Vdot : Inport  Port=3
  Bus Selector1 : BusSelector  OutputSignals=Tc,x_H2O,x_CO2,rho
  Bus Selector2 : BusSelector  OutputSignals=Tc,x_H2O,x_CO2,rho
  Demux5 : Demux  Outputs=2
  Fcn{1..4} (4 alike) : Fcn  Expr=u / (1+u)
  Gain : Gain  Gain=perc_Vdot_tot
  Gain{1,4..5,7} (4 alike) : Gain  Gain=-1
  Gain2 : Gain  Gain=0
  Ground{1..6,12..13} (8 alike) : Ground
  Mux1 : Mux  Inputs=[1 2 1 1 1 5 1 7]
  Mux2 : Mux  Inputs=[1 2 1 1 1 5 1 7]
  Mux3 : Mux  Inputs=2
  Mux6 : Mux  Inputs=2
  Product5 : Product  SaturateOnIntegerOverflow=on  InputSameDT=on  OutDataTypeStr=Inherit: Same as first input
  Product6 : Product  SaturateOnIntegerOverflow=on  InputSameDT=on  OutDataTypeStr=Inherit: Same as first input
  Product7 : Product  Inputs=3  SaturateOnIntegerOverflow=on  InputSameDT=on  OutDataTypeStr=Inherit: Same as first input
  Sum1 : Sum  Inputs=-+  SaturateOnIntegerOverflow=on  InputSameDT=on  OutDataTypeStr=Inherit: Same as first input
  Switch : Switch  Criteria=u2 > Threshold
  Switch1 : Switch  Criteria=u2 > Threshold
  cp : Constant  Value=1006.8
  h/s : Gain  Gain=1/3600
  "[S]_in" : Outport
  "[S]_out" : Outport  Port=2
  wires:
  Gain2/1 -> Mux2/1
  Ground6/1 -> Mux2/8
  Ground5/1 -> Mux2/6
  Gain5/1 -> Mux2/5
  Ground2/1 -> Mux2/2
  Gain7/1 -> Mux2/3
  Gain4/1 -> Mux2/4
  Ground3/1 -> Mux2/7
  Gain1/1 -> Mux1/3, Product7/2, Product5/1, Gain7/1  "massflow"
  h/s/1 -> Product6/1
  Vdot/1 -> Gain/1
  Sum1/1 -> Product7/1  "dT"
  Switch1/1 -> Product5/2
  Bus Selector2/2 -> Fcn2/1  "<x_H2O>"
  Bus Selector2/1 -> Sum1/2  "<Tc>"
  Demux5/1 -> Gain4/1, Mux1/4  "mdot_H2O"
  Demux5/2 -> Gain5/1, Mux1/5  "mdot_CO2"
  Ground13/1 -> Mux1/2
  Product7/1 -> Mux1/1, Gain2/1  "Qdot_air"
  Mux1/1 -> "[S]_in"/1
  Gain/1 -> h/s/1, Switch1/2, Switch/2
  Product6/1 -> Gain1/1
  Switch/1 -> Product6/2  "rho"
  Mux2/1 -> "[S]_out"/1
  Bus Selector2/3 -> Fcn1/1  "<x_CO2>"
  Product5/1 -> Demux5/1
  Ground12/1 -> Mux1/6
  Fcn2/1 -> Mux6/1
  Fcn1/1 -> Mux6/2
  Bus Selector1/1 -> Sum1/1  "<Tc>"
  "[AIB]_out"/1 -> Bus Selector2/1
  Ground1/1 -> Mux1/8
  Ground4/1 -> Mux1/7
  cp/1 -> Product7/3
  "[AIB]_in"/1 -> Bus Selector1/1
  Bus Selector1/4 -> Switch/1  "<rho>"
  Bus Selector2/4 -> Switch/3  "<rho>"
  Fcn4/1 -> Mux3/1
  Fcn3/1 -> Mux3/2
  Bus Selector1/2 -> Fcn4/1  "<x_H2O>"
  Bus Selector1/3 -> Fcn3/1  "<x_CO2>"
  Mux6/1 -> Switch1/3
  Mux3/1 -> Switch1/1
